simulink model "test"  (R2020a)
settings: Solver=VariableStepAuto  StartTime=0.0  StopTime=10.0  RelTol=1e-3
libraries: SignalEditorBlockLib x1
settings Model: Creator=Roland Varga  LastModifiedBy=Roland Varga

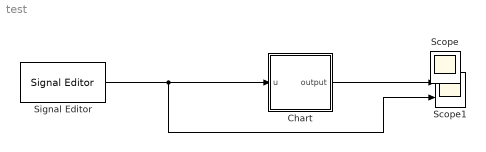
== system test ==
  Chart : Stateflow chart  TreatAsAtomicUnit=on
  Scope1 : Scope  NumInputPorts=2
  Signal Editor : SignalEditorBlockLib/Signal Editor  FileName=input_for_signaleditor.mat  ActiveScenario=Scenario  ActiveSignal=input  IsBus=off  OutputBusObjectStr=Bus: BusObject  SampleTime=0  Interpolate=off  ZeroCross=off  OutputAfterFinalValue=Setting to zero  Unit=inherit  PreserveSignalName=on
  Scope : Scope
  wires:
  Chart/1(output) -> Scope1/1
  Signal Editor/1 -> Scope1/2, Chart/1(u)

== stateflow chart test/Chart ==
  settings: stateMachineType=MOORE_MACHINE
  state init
    output = -2;
  state init1
    output = -1;
  init -> init1 : [u==1]
  (default) -> init
  init1 -> init : [u==0]
  data: u input; output output
